simulink model "PI_delta_fix"  (R2017b)
settings: Solver=ode3  StartTime=0.0  StopTime=50  FixedStep=DT  MaxStep=DT  RelTol=1e-3  EnableMultiTasking=on
undefined symbols (not defined in the file): deltaapc, dPchLim, NDOF, NumOuts, OutList, PC_KI, PC_KK, PC_KP, PchLim, Pitch_0_rad, Prat, q_init, qdot_init, strmatch, Trat, Ts, VSspeeds, VStorques, WT5MWrotor
libraries: simulink_extras x1, wturbine_lib x1
settings Model: Creator=fbianchi  LastModifiedBy=Bernabé
settings SolverCC: ZeroCrossAlgorithm=Adaptive
settings DataIOCC: FinalStateName=estados  InitialState=SimState  LimitDataPoints=on  SaveFinalState=on  SaveCompleteFinalSimState=on  SaveFormat=Array  SignalLoggingSaveFormat=ModelDataLogs  SaveOutput=off  SaveTime=off  SignalLoggingName=sigsOut
settings OptimizationCC: ExpressionDepthLimit=2147483647  LifeSpan=inf
settings DebuggingCC: SaveWithParameterizedLinksMsg=none  UnderspecifiedInitializationDetection=Classic  MergeDetectMultiDrivingBlocksExec=none  SignalResolutionControl=TryResolveAllWithWarning  IgnoredZcDiagnostic=none  MultiTaskDSMMsg=warning  MultiTaskCondExecSysMsg=none  FcnCallInpInsideContextMsg=warning  StateNameClashWarn=warning  StrictBusMsg=None  SFUnexpectedBacktrackingDiag=warning  SFNoUnconditionalDefaultTransitionDiag=warning  SFExecutionAtInitializationDiag=none
settings HardwareCC: ProdBitPerPointer=32  ProdBitPerSizeT=32  ProdBitPerPtrDiffT=32  ProdLargestAtomicFloat=None  ProdIntDivRoundTo=Undefined  ProdEndianess=Unspecified  ProdWordSize=32  ProdHWDeviceType=32-bit Generic  TargetUnknown=on
settings ModelReferenceCC: PropagateSignalLabelsOutOfModel=off
settings CodeAppCC: StateflowObjectComments=on
settings GRTTargetCC: TargetLangStandard=C89/C90 (ANSI)  GeneratePreprocessorConditionals=Disable all  CombineOutputUpdateFcns=off  GRTInterface=on
settings ConfigComp: CovMetricSettings=dw  CovHtmlReporting=on  CovSaveCumulativeToWorkspaceVar=on  CovSaveSingleToWorkspaceVar=on  CovExternalEMLEnable=off

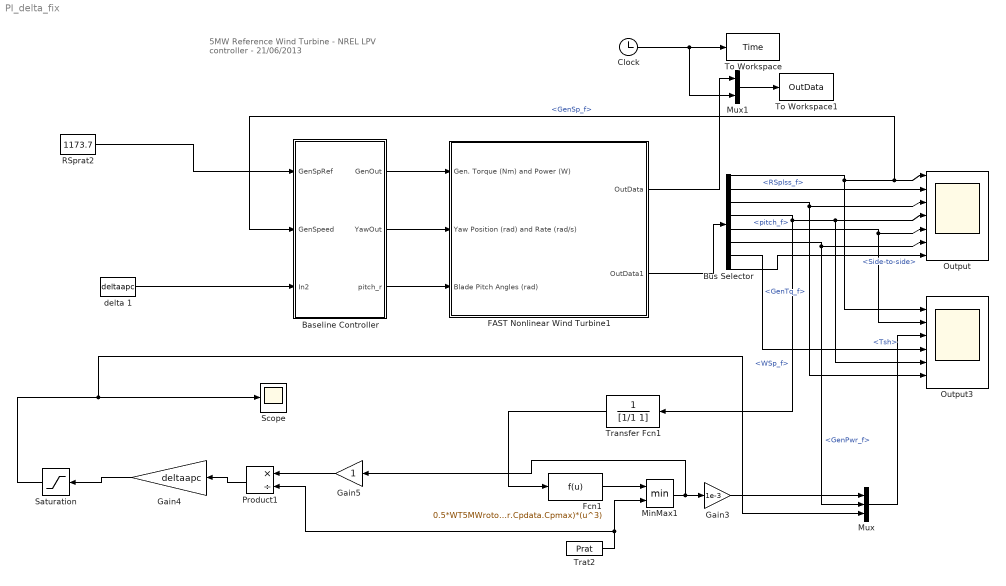
== system PI_delta_fix ==
  note: 5MW Reference Wind Turbine - NREL
      | LPV controller
      |  - 21/06/2013
  Baseline Controller : Subsystem
  Bus Selector : BusSelector  OutputSignals=GenSp_f,RSplss_f,GenTq_f,WSp_f,pitch_f,GenPwr_f,Tsh,Side-to-side
  Clock : Clock
  FAST Nonlinear Wind Turbine1 : Subsystem  mask(FAST Nonlinear Wind Turbine){}
      mask help: This block contains the FAST S-Function and blocks that integrate the DOF accelerations to get velocities and displacements.
      mask init:
      | clear FAST_SFunc
  Fcn1 : Fcn  Expr=0.5*WT5MWrotor.rho*(WT5MWrotor.R^2*pi)*(WT5MWrotor.Cpdata.Cpmax)*(u^3)
  Gain3 : Gain  Gain=1e-3
  Gain4 : Gain  Gain=deltaapc
  Gain5 : Gain
  MinMax1 : MinMax  Inputs=2
  Mux : Mux  Inputs=3
  Mux1 : Mux  Inputs=2
  Output : Scope  NumInputPorts=7
  Output3 : Scope  NumInputPorts=6
  Product1 : Product  Inputs=*/  RndMeth=Zero
  RSprat2 : Constant  Value=1173.7
  Saturation : Saturate  UpperLimit=100  LowerLimit=30
  Scope : Scope
  To Workspace : ToWorkspace  VariableName=Time  SampleTime=-1
  To Workspace1 : ToWorkspace  VariableName=OutData  SampleTime=-1
  Transfer Fcn1 : TransferFcn  Denominator=[1/1 1]
  Trat2 : Constant  Value=Prat
  delta 1 : Constant  Value=deltaapc
  wires:
  Bus Selector/2 -> Output/2  "<RSplss_f>"
  Bus Selector/3 -> Output3/6, Output/3  "<GenTq_f>"
  Bus Selector/5 -> Output3/2, Output/5  "<pitch_f>"
  Bus Selector/6 -> Mux/2, Output/6  "<GenPwr_f>"
  Bus Selector/1 -> Output3/1, Baseline Controller/2(GenSpeed), Output/1  "<GenSp_f>"
  FAST Nonlinear Wind Turbine1/2(OutData1) -> Bus Selector/1
  Bus Selector/7 -> Output3/4  "<Tsh>"
  Bus Selector/4 -> Transfer Fcn1/1, Output3/5, Output/4  "<WSp_f>"
  Fcn1/1 -> MinMax1/1
  Trat2/1 -> Product1/2, MinMax1/2
  MinMax1/1 -> Gain5/1, Gain3/1
  Gain3/1 -> Mux/1
  Mux/1 -> Output3/3
  RSprat2/1 -> Baseline Controller/1(GenSpRef)
  Transfer Fcn1/1 -> Fcn1/1
  Saturation/1 -> Mux/3, Scope/1
  Product1/1 -> Gain4/1
  Gain5/1 -> Product1/1
  Gain4/1 -> Saturation/1
  delta 1/1 -> Baseline Controller/3(In2)
  Mux1/1 -> To Workspace1/1
  FAST Nonlinear Wind Turbine1/1(OutData) -> Mux1/1
  Clock/1 -> Mux1/2, To Workspace/1
  Baseline Controller/2(YawOut) -> FAST Nonlinear Wind Turbine1/2(Yaw Position (rad) and Rate (rad/s))
  Baseline Controller/3(pitch_r) -> FAST Nonlinear Wind Turbine1/3(Blade Pitch Angles (rad))
  Baseline Controller/1(GenOut) -> FAST Nonlinear Wind Turbine1/1(Gen. Torque (Nm) and Power (W))
  Bus Selector/8 -> Output/7  "<Side-to-side>"

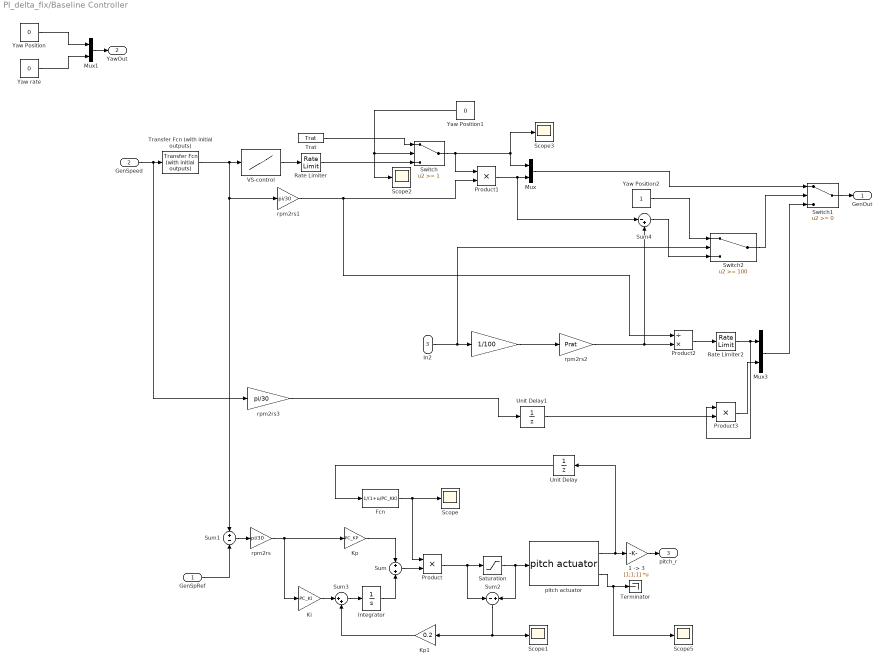
== system PI_delta_fix/Baseline Controller ==
  GenSpRef : Inport
  GenSpeed : Inport  Port=2
  In2 : Inport  Port=3
  " " : Gain  Gain=1/100
  "1 -> 3" : Gain  Gain=[1;1;1]  Multiplication=Matrix(K*u)
  Fcn : Fcn  Expr=1/(1+u/PC_KK)
  Integrator : Integrator  InitialCondition=Pitch_0_rad
  Ki : Gain  Gain=PC_KI
  Kp : Gain  Gain=PC_KP
  Kp1 : Gain  Gain=0.2
  Mux : Mux  Inputs=2
  Mux1 : Mux  Inputs=2
  Mux3 : Mux  Inputs=2
  Product : Product  RndMeth=Zero
  Product1 : Product  RndMeth=Zero
  Product2 : Product  Inputs=/*  RndMeth=Zero
  Product3 : Product  Inputs=**  RndMeth=Zero
  Rate Limiter : RateLimiter  RisingSlewLimit=15000  FallingSlewLimit=-15000  SampleTimeMode=inherited
  Rate Limiter2 : RateLimiter  RisingSlewLimit=15000  FallingSlewLimit=-15000
  Saturation : Saturate  UpperLimit=PchLim(2)*pi/180  LowerLimit=PchLim(1)*pi/180
  Scope{,1..3,5} (5 alike) : Scope
  Sum : Sum
  Sum1 : Sum  Inputs=+-
  Sum2 : Sum  Inputs=-+
  Sum3 : Sum  Inputs=|++
  Sum4 : Sum  Inputs=|-+
  Switch : Switch  Threshold=1
  Switch1 : Switch
  Switch2 : Switch  Threshold=100
  Terminator : Terminator
  Transfer Fcn (with initial outputs) : simulink_extras/Additional Linear/Transfer Fcn (with initial outputs)  N=[1]  D="[1/1.57  1]"  Y0=1173.7  U0=0
  Trat : Constant  Value=Trat
  Unit Delay : UnitDelay  InitialCondition=Pitch_0_rad  SampleTime=Ts
  Unit Delay1 : UnitDelay  InitialCondition=Pitch_0_rad  SampleTime=Ts
  VS-control : Lookup_n-D  NumberOfTableDimensions=1  BreakpointsForDimension1=VSspeeds  Table=VStorques  RndMeth=Simplest  InputSameDT=on
  Yaw Position : Constant  Value=0
  Yaw Position1 : Constant  Value=0
  Yaw Position2 : Constant
  Yaw rate : Constant  Value=0
  pitch actuator : wturbine_lib/pitch actuator  tau=1/3  pitch_lim=PchLim*pi/180  pitch_rate_lim=dPchLim*pi/180  pitch_0=Pitch_0_rad
  rpm2rs : Gain  Gain=pi/30
  rpm2rs1 : Gain  Gain=pi/30
  rpm2rs2 : Gain  Gain=Prat
  rpm2rs3 : Gain  Gain=pi/30
  GenOut : Outport
  YawOut : Outport  Port=2
  pitch_r : Outport  Port=3
  wires:
  Ki/1 -> Sum3/1
  Sum3/1 -> Integrator/1
  rpm2rs/1 -> Kp/1, Ki/1
  Kp/1 -> Sum/1
  Integrator/1 -> Sum/2
  Yaw Position1/1 -> Switch/2, Scope2/1
  Switch/1 -> Product1/1, Scope3/1, Mux/1
  Kp1/1 -> Sum3/2
  Sum2/1 -> Kp1/1, Scope1/1
  Saturation/1 -> pitch actuator/1, Sum2/2
  Product/1 -> Saturation/1, Sum2/1
  Trat/1 -> Switch/1
  Rate Limiter/1 -> Switch/3
  Unit Delay/1 -> Fcn/1
  Transfer Fcn (with initial outputs)/1 -> VS-control/1, rpm2rs1/1, Sum1/1
  GenSpRef/1 -> Sum1/2
  Sum1/1 -> rpm2rs/1
  Yaw rate/1 -> Mux1/2
  Yaw Position/1 -> Mux1/1
  Mux1/1 -> YawOut/1
  GenSpeed/1 -> rpm2rs3/1, Transfer Fcn (with initial outputs)/1
  VS-control/1 -> Rate Limiter/1
  Mux/1 -> Switch1/1
  pitch actuator/2 -> Scope5/1, Terminator/1
  pitch actuator/1 -> Unit Delay/1, "1 -> 3"/1
  "1 -> 3"/1 -> pitch_r/1
  Fcn/1 -> Product/1, Scope/1
  Sum/1 -> Product/2
  Product1/1 -> Sum4/1, Mux/2
  Product2/1 -> Rate Limiter2/1
  " "/1 -> rpm2rs2/1
  Mux3/1 -> Switch1/3
  Rate Limiter2/1 -> Mux3/1, Product3/1
  In2/1 -> Switch2/2, " "/1
  rpm2rs1/1 -> Product2/1, Product1/2
  rpm2rs2/1 -> Product2/2, Sum4/2
  Product3/1 -> Mux3/2
  Switch1/1 -> GenOut/1
  Sum4/1 -> Switch2/3
  Switch2/1 -> Switch1/2
  Yaw Position2/1 -> Switch2/1
  rpm2rs3/1 -> Unit Delay1/1
  Unit Delay1/1 -> Product3/2

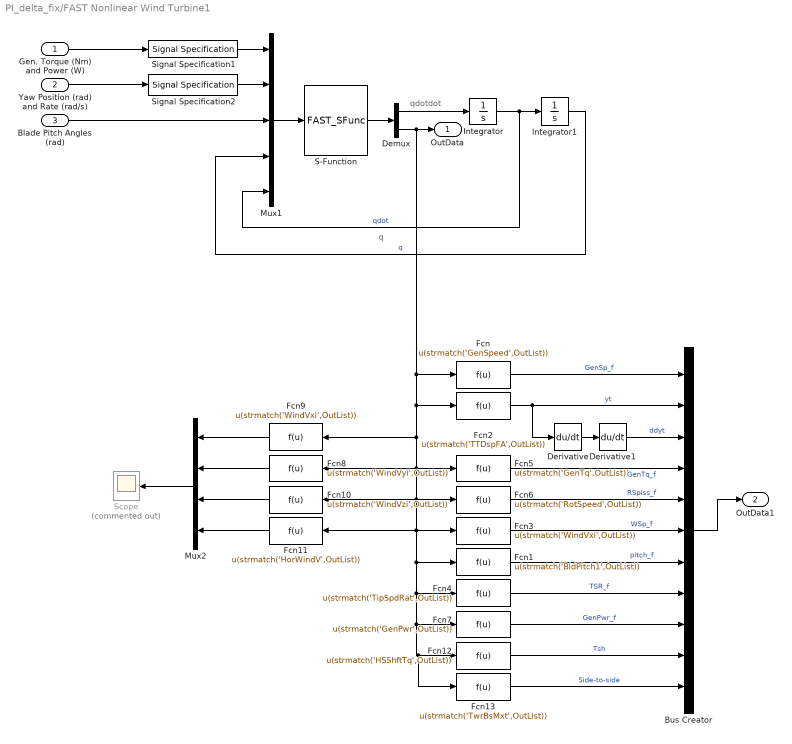
== system PI_delta_fix/FAST Nonlinear Wind Turbine1 ==
  note: qdotdot
  note: q
  Gen. Torque (Nm) and Power (W) : Inport
  Yaw Position (rad) and Rate (rad/s) : Inport  Port=2
  Blade Pitch Angles (rad) : Inport  Port=3
  Bus Creator : BusCreator  Inputs=11
  Demux : Demux  Outputs=[NDOF, NumOuts]
  Derivative : Derivative
  Derivative1 : Derivative
  Fcn : Fcn  Expr=u(strmatch('GenSpeed',OutList))
  Fcn1 : Fcn  Expr=u(strmatch('BldPitch1',OutList))
  Fcn10 : Fcn  Expr=u(strmatch('WindVzi',OutList))
  Fcn11 : Fcn  Expr=u(strmatch('HorWindV',OutList))
  Fcn12 : Fcn  Expr=u(strmatch('HSShftTq',OutList))
  Fcn13 : Fcn  Expr=u(strmatch('TwrBsMxt',OutList))
  Fcn2 : Fcn  Expr=u(strmatch('TTDspFA',OutList))
  Fcn3 : Fcn  Expr=u(strmatch('WindVxi',OutList))
  Fcn4 : Fcn  Expr=u(strmatch('TipSpdRat',OutList))
  Fcn5 : Fcn  Expr=u(strmatch('GenTq',OutList))
  Fcn6 : Fcn  Expr=u(strmatch('RotSpeed',OutList))
  Fcn7 : Fcn  Expr=u(strmatch('GenPwr',OutList))
  Fcn8 : Fcn  Expr=u(strmatch('WindVyi',OutList))
  Fcn9 : Fcn  Expr=u(strmatch('WindVxi',OutList))
  Integrator : Integrator  InitialCondition=qdot_init
  Integrator1 : Integrator  InitialCondition=q_init
  Mux1 : Mux  Inputs=5
  Mux2 : Mux
  S-Function : S-Function  FunctionName=FAST_SFunc  SFunctionDeploymentMode=off  EnableBusSupport=off
  Scope : Scope  Commented=on
  Signal Specification1 : SignalSpecification  OutDataTypeStr=double  Dimensions=2
  Signal Specification2 : SignalSpecification  OutDataTypeStr=double  Dimensions=2
  OutData : Outport
  OutData1 : Outport  Port=2
  wires:
  Integrator/1 -> Integrator1/1, Mux1/5  "qdot"
  Gen. Torque (Nm) and Power (W)/1 -> Signal Specification1/1
  S-Function/1 -> Demux/1
  Demux/1 -> Integrator/1
  Mux1/1 -> S-Function/1
  Blade Pitch Angles (rad)/1 -> Mux1/3
  Yaw Position (rad) and Rate (rad/s)/1 -> Signal Specification2/1
  Integrator1/1 -> Mux1/4  "q"
  Signal Specification1/1 -> Mux1/1
  Signal Specification2/1 -> Mux1/2
  Derivative1/1 -> Bus Creator/3  "ddyt"
  Fcn3/1 -> Bus Creator/6  "WSp_f"
  Mux2/1 -> Scope/1
  Fcn2/1 -> Derivative/1, Bus Creator/2  "yt"
  Fcn6/1 -> Bus Creator/5  "RSplss_f"
  Demux/2 -> Fcn13/1, Fcn12/1, Fcn7/1, Fcn4/1, Fcn1/1, Fcn11/1, Fcn3/1, Fcn10/1, Fcn6/1, Fcn8/1, Fcn5/1, Fcn9/1, Fcn2/1, Fcn/1, OutData/1
  Fcn11/1 -> Mux2/4
  Fcn/1 -> Bus Creator/1  "GenSp_f"
  Fcn12/1 -> Bus Creator/10  "Tsh"
  Derivative/1 -> Derivative1/1
  Bus Creator/1 -> OutData1/1
  Fcn1/1 -> Bus Creator/7  "pitch_f"
  Fcn4/1 -> Bus Creator/8  "TSR_f"
  Fcn7/1 -> Bus Creator/9  "GenPwr_f"
  Fcn10/1 -> Mux2/3
  Fcn5/1 -> Bus Creator/4  "GenTq_f"
  Fcn9/1 -> Mux2/1
  Fcn8/1 -> Mux2/2
  Fcn13/1 -> Bus Creator/11  "Side-to-side"
